simulink model "teste_bloco_atenuacao"  (R2014a)
settings: Solver=ode3  StartTime=0.0  StopTime=0.01  RelTol=1e-3
libraries: simulink x4, dspmathops x2, dspsigops x1
settings Model: Creator=andre  LastModifiedBy=andre
settings DebuggingCC: SolverPrmCheckMsg=none

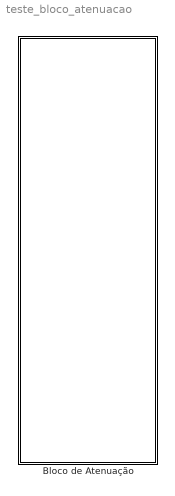
== system teste_bloco_atenuacao ==
  Bloco de Atenuação : Subsystem

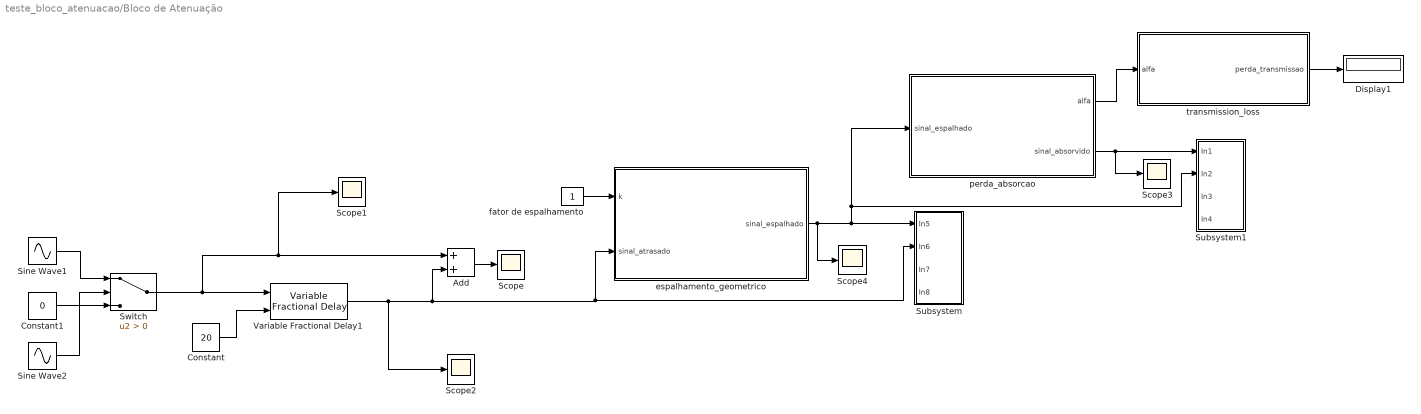
== system teste_bloco_atenuacao/Bloco de Atenuação ==
  Add : Sum
  Constant : Constant  Value=20  SampleTime=0
  Constant1 : Constant  Value=0
  Display1 : Display
      settings: Decimation=2
  Scope{,1..4} (5 alike) : Scope
      Scope settings: SampleTime=1000
      Scope1 settings: SampleTime=1000
      Scope2 settings: SaveName=ScopeData2  SampleTime=1000
      Scope3 settings: SaveName=ScopeData3  SampleTime=1000
      Scope4 settings: SaveName=ScopeData4  SampleTime=1000
  Sine Wave1 : Sin  SineType=Sample based  Amplitude=3  Frequency=100  Samples=20  SampleTime=1/20000
  Sine Wave2 : Sin  SampleTime=1/20000
  Subsystem : Subsystem
  Subsystem1 : Subsystem
  Switch : Switch  Criteria=u2 > Threshold
  Variable Fractional Delay1 : dspsigops/Variable Fractional Delay  mode=OBSOLETE  modeActive=Linear  dmax=10000  InputProcessing=Columns as channels (frame based)  L=4  FarrowL=4  R=10  alpha=1  ic=0  fallbackFIR=Clip to the minimum value necessary for centered kernel  fallbackFarrow=Clip to the minimum value necessary for centered kernel  noDFT=off  roundingMode=Zero  overflowMode=off
  espalhamento_geometrico : MATLAB Function  TreatAsAtomicUnit=on
  fator de espalhamento : Constant
  perda_absorcao : MATLAB Function  TreatAsAtomicUnit=on
  transmission_loss : MATLAB Function  TreatAsAtomicUnit=on
  wires:
  fator de espalhamento/1 -> espalhamento_geometrico/1(k)
  Constant/1 -> Variable Fractional Delay1/2
  Variable Fractional Delay1/1 -> espalhamento_geometrico/2(sinal_atrasado), Subsystem/2(In6), Add/2, Scope2/1
  Sine Wave1/1 -> Switch/1
  Sine Wave2/1 -> Switch/2
  Constant1/1 -> Switch/3
  Switch/1 -> Add/1, Scope1/1, Variable Fractional Delay1/1
  Add/1 -> Scope/1
  perda_absorcao/2(sinal_absorvido) -> Scope3/1, Subsystem1/1(In1)
  transmission_loss/1(perda_transmissao) -> Display1/1
  perda_absorcao/1(alfa) -> transmission_loss/1(alfa)
  espalhamento_geometrico/1(sinal_espalhado) -> Scope4/1, perda_absorcao/1(sinal_espalhado), Subsystem1/2(In2), Subsystem/1(In5)

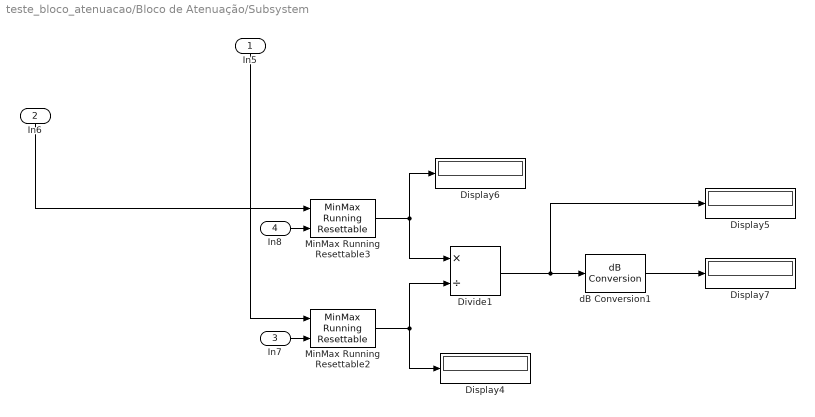
== system teste_bloco_atenuacao/Bloco de Atenuação/Subsystem ==
  In5 : Inport
  In6 : Inport  Port=2
  In7 : Inport  Port=3
  In8 : Inport  Port=4
  Display{4..7} (4 alike) : Display
      Display5 settings: Decimation=2
      Display7 settings: Decimation=2
  Divide1 : Product  Inputs=*/
  MinMax Running Resettable2 : simulink/Math Operations/MinMax Running Resettable  Function=max  vinit=0.0
  MinMax Running Resettable3 : simulink/Math Operations/MinMax Running Resettable  Function=max  vinit=0.0
  dB Conversion1 : dspmathops/dB Conversion  dBtype=dB  intype=Amplitude  R=1  fuzz=off
  wires:
  In8/1 -> MinMax Running Resettable3/2
  In6/1 -> MinMax Running Resettable3/1
  In5/1 -> MinMax Running Resettable2/1
  In7/1 -> MinMax Running Resettable2/2
  dB Conversion1/1 -> Display7/1
  MinMax Running Resettable3/1 -> Display6/1, Divide1/1
  MinMax Running Resettable2/1 -> Display4/1, Divide1/2
  Divide1/1 -> dB Conversion1/1, Display5/1

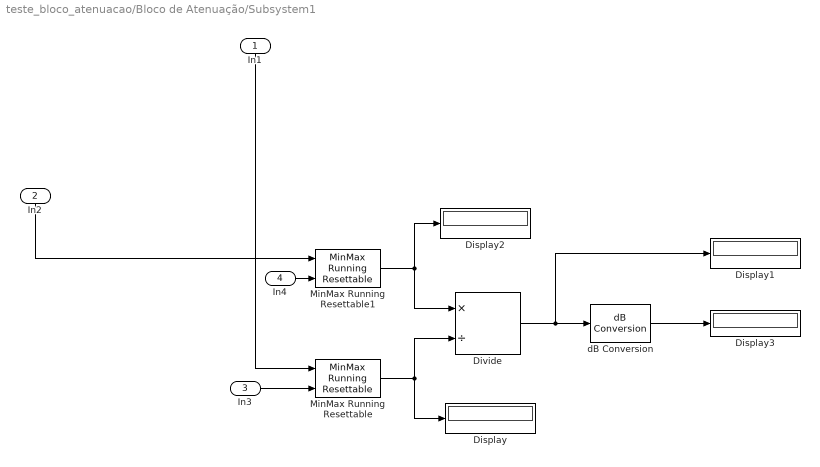
== system teste_bloco_atenuacao/Bloco de Atenuação/Subsystem1 ==
  In1 : Inport
  In2 : Inport  Port=2
  In3 : Inport  Port=3
  In4 : Inport  Port=4
  Display{,1..3} (4 alike) : Display
      Display1 settings: Decimation=2
      Display3 settings: Decimation=2
  Divide : Product  Inputs=*/
  MinMax Running Resettable : simulink/Math Operations/MinMax Running Resettable  Function=max  vinit=0.0
  MinMax Running Resettable1 : simulink/Math Operations/MinMax Running Resettable  Function=max  vinit=0.0
  dB Conversion : dspmathops/dB Conversion  dBtype=dB  intype=Amplitude  R=1  fuzz=off
  wires:
  In4/1 -> MinMax Running Resettable1/2
  In1/1 -> MinMax Running Resettable/1
  In3/1 -> MinMax Running Resettable/2
  dB Conversion/1 -> Display3/1
  MinMax Running Resettable1/1 -> Display2/1, Divide/1
  MinMax Running Resettable/1 -> Display/1, Divide/2
  Divide/1 -> dB Conversion/1, Display1/1
  In2/1 -> MinMax Running Resettable1/1

== matlab function teste_bloco_atenuacao/Bloco de Atenuação/transmission_loss ==
  data: alfa input; perda_transmissao output
function perda_transmissao  = transmission_loss(alfa)
%--------------------------------------------------------------------------
%A equação que define a perda de transmissão para ambientes de  aguas rasas
%é dada pela expressão:
% TL = 10 log10*r + alfa*r * 10^-3  (dB/km) , onde:
% r = caminho = distância em metros
% alfa = coeficiente de absorção 
%--------------------------------------------------------------------------
caminho = 6;

perda_transmissao = 10*log10(caminho) + alfa * caminho * 10^-3;

== matlab function teste_bloco_atenuacao/Bloco de Atenuação/perda_absorcao ==
  data: alfa output; sinal_espalhado input; sinal_absorvido output
function [alfa,sinal_absorvido] = perda_absorcao(sinal_espalhado)
% Calcular o coeficeinte de absorção (a)
% Calcular a perda por absorção

% Parâmetros Ambientais
T = 30;                 % Temperatura da água
S = 35;                 % Salinidade da água do mar do litoral brasileiro (1 milligram/liter [mg/L] = 1,000000002 part/million [ppm])
pH = 7.8;               % Acidez da água

% Parâmetro da Geometria do Aquário
D = 0.003;              % Profundidade em km
caminho = 6;            % Comprimento do aquário em metros
frequencia = 19.670;     % em kHz

%c = 1412 + 3.21*T + 1.19*S + 0.0167*D;  % velocidade do som em metros/segundos

%Valores dos parâmetros Para o primeiro Coeficiente de Absorção(alfa)  
f1 = 0.78 * sqrt(S/35) * (exp(T/26));    % Ácido Bórico
f2 = 42 * (exp(T/17));                   % Sulfato de Magnésio

%f1 = 2.8 * (S/35)^0.5 * 10^[4-1245/(273+T)];        % frequencia (kHz) de relaxação para o Ácido Bórico
%f2 = 8.17*10^[8-1990/(273+T)] / 1 + 0.0018*(S-35);  % frequencia (kHz) de relaxação para o Sulfato de Magnésio

%A1 = (8.68/c)*10^(0.78*pH-5);       % componente do Ácido Bórico para água do mar
%P1 = 1;     % pressão da profundidade para o ádico bórico na água do mar

%A2 = 21.44 * (S/c) * (1 + 0.025 * T);       % componente do Sulfato de Magnésio para água do mar
%P2 = 1 - 1.37 * 10^-4 * D + 6.2 * 10 - 9 * D^2;     % pressão da profundidade para o sulfato de magnésio na água do mar

% Componente da Viscosidade (água pura) na água do mar
%A3 = 4.937 * 10^-4 - 2.59 * 10^-5 * T + 9.11 * 10^-7 * T^2 - 1.5 * 10^-8 * T^3; % para T <= 20°C
%A3 = 3.964 * 10^-4 - 1.146 * 10^-5 * T + 1.45 * 10^-7 * T^2 - 6.5 * 10^-10 * T^3; % para T >= 20°C
%P3 = 1 - 3.83 * 10^-5 * D + 4.9 * 10^-10 * D^2;     % pressão da profundidade para a viscosidade(água pura) na água do mar

%--------------------------------------------------------------------------
% Coeficiente de Absorção(alfa). Escolher o tipo de expressão que depende 
% diretamente da frequencia do sinal.
%--------------------------------------------------------------------------

alfa = ((0.106 * (f1 * frequencia^2) * exp((pH - 8) / 0.56)) /...
    (f1^2 + frequencia^2)) + ((0.52 * (1 + (T / 43)) * (S / 35) *...
    (f2 * frequencia^2) * exp(-(D / 6))) / (f2^2 + frequencia^2)) +...
    (0.00049 * (frequencia^2) * (exp(-(T/27 + D/17))))

%--------------------------------------------------------------------------
% Para frequências acima de algumas centenas de Hz usar o coeficiente de 
% absorção(alfa) da expressão de Thorp [Principles of Underwater Sound]

% alfa = (A1 * P1 * f1 * frequencia^2) / (frequencia^2 + f1^2) +...
%     (A2 * P2 * f2 * frequencia^2) / (frequencia^2 + f2^2) + A3 * P3 * frequencia^2;

%--------------------------------------------------------------------------
% Para frequências baixas usar fórmula do coeficiente de absorção(alfa) da 
% referência [Fundamentals of Ocean Acoustics]:

% alfa = 0.002 + 0.11 * frequencia^2 / 1 + frequencia^2 + 0.011 * frequencia^2;
%--------------------------------------------------------------------------
% Convertendo o coeficiente de absorção(alfa) de km para m:
%alfa = alfa * 10^-3    

%--------------------------------------------------------------------------
% Perda_absorção = 10log(a)*r (dB)
% Esse coeficiente varia linerarmente com a faixa r em quilômetros para um
% dado valor de frequência
%--------------------------------------------------------------------------

perda_absorcao = 10*log10(alfa)*caminho

%-------------------------------------------------------------------------
% Equação para o espalhamento do sinal utilizando a razao normal de ganho
% em que G=(Pout/Pin)<1
% in = sinal_espalhado*10^(atenuacao/10) 
%-------------------------------------------------------------------------

sinal_absorvido = sinal_espalhado.*(10^(-perda_absorcao/10));

%-------------------------------------------------------------------------
% Equação para atenuação do sinal (G(db) < 0)
% G(dB) = Pout(dB) - Pin(dB)
% G(dB) = sinal_atenuado - sinal_espalhado 
%------------------------------------------------------------------------

== matlab function teste_bloco_atenuacao/Bloco de Atenuação/espalhamento_geometrico ==
  data: k input; sinal_atrasado input; sinal_espalhado output
function sinal_espalhado  = espalhamento_geometrico(k,sinal_atrasado)

%a perda por espalhamento geométrico é calculado a partir da equação da
%dissertação:   perda_espalhamento = k * 10log(r); 
%   k = fator de espalhamento
%   caminhos = distância em metros que o sinal percorre ao longo da propagação

caminho = 6;
%-------------------------------------------------------------------------
%Equação para cálculo da perda por espalhamento geométrico (Spreading Loss)
%-------------------------------------------------------------------------
perda_espalhamento = k * 10*log10(caminho)

%-------------------------------------------------------------------------
% Equação para o espalhamento do sinal utilizando a razao normal de ganho
% em que G=(Pout/Pin)<1
% in = sinal_atrasado*10^(espalhamento/10)
%-------------------------------------------------------------------------
sinal_espalhado = sinal_atrasado.*(10^(-perda_espalhamento/10));
